simulink model "Simulink"  (R2020b)
settings: Solver=VariableStepAuto  StartTime=0.0  StopTime=5  RelTol=1e-3
values from neighbouring files (symbols this model uses):
  d1 = 0.01    [Parameters.m]    (also in SYS.mat)
  d2 = 0.01    [Parameters.m]    (also in SYS.mat)
  g = 9.82    [Parameters.m]    (also in SYS.mat = 0.666666666667)
  L = 1    [Parameters.m]    (also in SYS.mat)
  mc = 1.5    [Parameters.m]    (also in SYS.mat)
  mp = 0.5    [Parameters.m]    (also in SYS.mat)
libraries: cstblocks x1
settings Model: Creator=bhuva  LastModifiedBy=bhuva

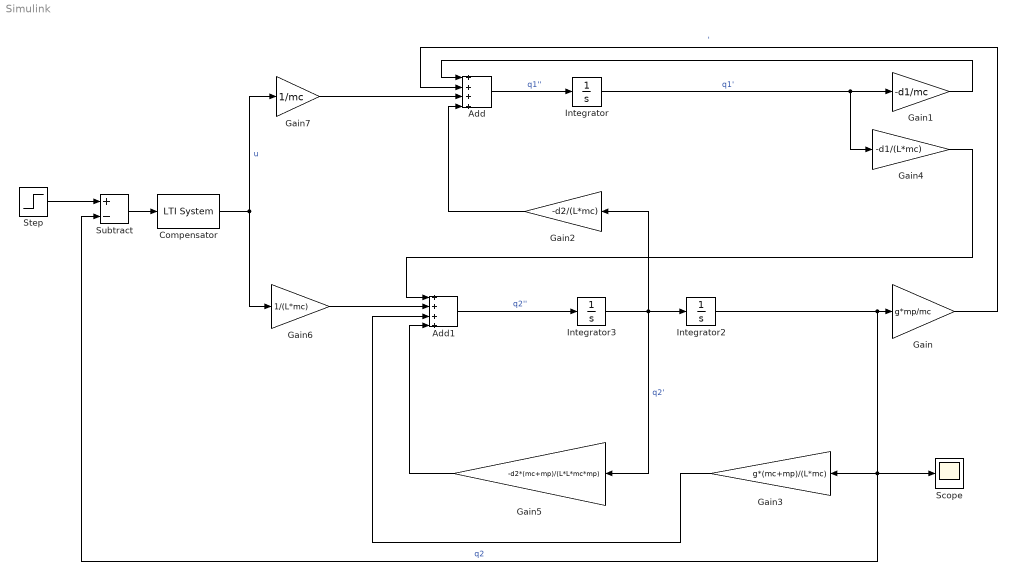
== system Simulink ==
  Add : Sum  Inputs=++++
  Add1 : Sum  Inputs=++++
  Compensator : cstblocks/LTI System  sys=C  IC=[]
  Gain : Gain  Gain=g*mp/mc
  Gain1 : Gain  Gain=-d1/mc
  Gain2 : Gain  Gain=-d2/(L*mc)
  Gain3 : Gain  Gain=g*(mc+mp)/(L*mc)
  Gain4 : Gain  Gain=-d1/(L*mc)
  Gain5 : Gain  Gain=-d2*(mc+mp)/(L*L*mc*mp)
  Gain6 : Gain  Gain=1/(L*mc)
  Gain7 : Gain  Gain=1/mc
  Integrator : Integrator
  Integrator2 : Integrator
  Integrator3 : Integrator
  Scope : Scope
  Step : Step  Time=0  SampleTime=0
  Subtract : Sum  Inputs=+-
  wires:
  Integrator/1 -> Gain1/1, Gain4/1  "q1'"
  Integrator3/1 -> Gain2/1, Integrator2/1, Gain5/1  "q2'"
  Gain/1 -> Add/2  "'"
  Add1/1 -> Integrator3/1  "q2''"
  Integrator2/1 -> Scope/1, Gain3/1, Subtract/2, Gain/1  "q2"
  Add/1 -> Integrator/1  "q1''"
  Gain1/1 -> Add/1
  Gain2/1 -> Add/4
  Gain5/1 -> Add1/4
  Gain4/1 -> Add1/1
  Gain3/1 -> Add1/3
  Gain7/1 -> Add/3
  Gain6/1 -> Add1/2
  Subtract/1 -> Compensator/1
  Step/1 -> Subtract/1
  Compensator/1 -> Gain6/1, Gain7/1  "u"
